simulink model "NeuralNetworkAdaptiveControl_Example"  (R2019a)
settings: Solver=VariableStepAuto  StartTime=0.0  StopTime=10.0  RelTol=1e-3
InitFcn:
  | ini_file
values from neighbouring files (symbols this model uses):
  gamma = 3    [ini_file_HW.m]
  wn = 3    [ini_file_HW.m]
  zeta = 1    [ini_file_HW.m]
undefined symbols (not defined in the file or in its folder): sigbuilder_block
settings Model: Creator=0629w  LastModifiedBy=0629w

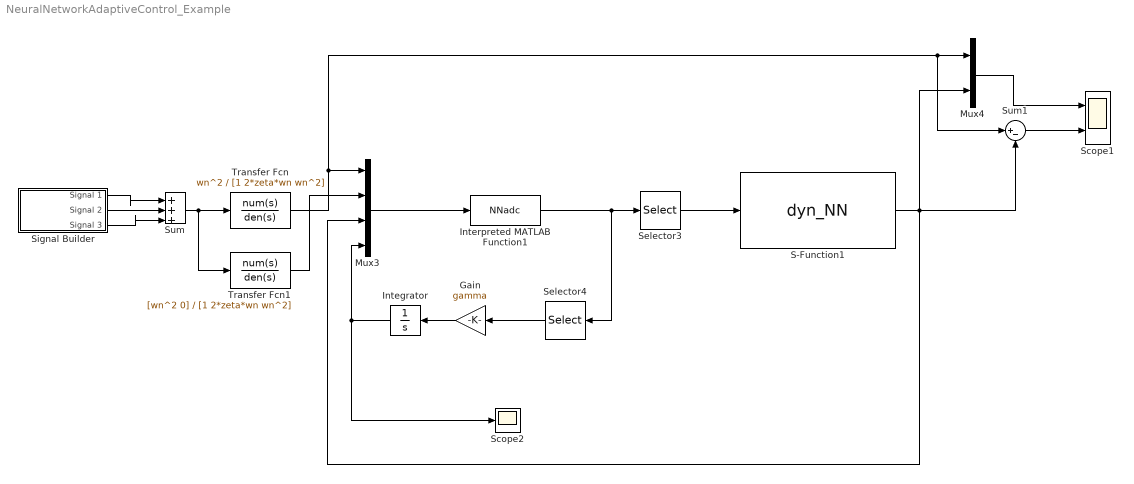
== system NeuralNetworkAdaptiveControl_Example ==
  Gain : Gain  Gain=gamma
  Integrator : Integrator
  Interpreted MATLAB Function1 : MATLABFcn  MATLABFcn=NNadc  OutputDimensions=3
  Mux3 : Mux
  Mux4 : Mux  Inputs=2
  S-Function1 : S-Function  FunctionName=dyn_NN  SFunctionDeploymentMode=off  EnableBusSupport=off
  Scope1 : Scope  NumInputPorts=2
  Scope2 : Scope
  Selector3 : Selector  InputPortWidth=3  IndexOptions=Index vector (dialog)  Indices=[1]  OutputSizes=1
  Selector4 : Selector  InputPortWidth=3  IndexOptions=Index vector (dialog)  Indices=[2 3]  OutputSizes=1
  Signal Builder : Subsystem  Tag=STV Subsys  LoadFcn=sigbuilder_block('load');  StartFcn=sigbuilder_block('start');  StopFcn=sigbuilder_block('stop');  ClipboardFcn=sigbuilder_block('clipboard');  mask(Sigbuilder block){tuvar=[0:10]}
      mask help: Simulink:masks:SigbuilderBlock_MD
      mask init:
      | if ~strcmp(get_param(bdroot(gcbh),'SimulationStatus'),'stopped') tuvar = sigbuilder_block('maskInit'); end
      settings: CopyFcn=sigbuilder_block('copy');  DeleteFcn=sigbuilder_block('delete');  ModelCloseFcn=sigbuilder_block('modelClose');  PreSaveFcn=sigbuilder_block('preSave');  PauseFcn=sigbuilder_block('pause');  ContinueFcn=sigbuilder_block('continue');  NameChangeFcn=sigbuilder_block('namechange');  OpenFcn=sigbuilder_block('open',[-192 38.25 1188 545.25 ]);  CloseFcn=sigbuilder_block('close');
      mask Display: plot(0, 0, 100, 100,[2, 2, 32, 32, 2], [68, 8, 8, 68, 68],[32, 2], [38, 38], [32, 19, 2],[53, 60, 44], [32, 17, 17, 2],[16, 16, 31, 31]);txt = getActiveGroup(gcbh);text(2, 100, txt,'verticalAlignment', 'top');
  Sum : Sum  Inputs=|+++
  Sum1 : Sum  Inputs=|+-
  Transfer Fcn : TransferFcn  Numerator=wn^2  Denominator=[1 2*zeta*wn wn^2]
  Transfer Fcn1 : TransferFcn  Numerator=[wn^2 0]  Denominator=[1 2*zeta*wn wn^2]
  wires:
  Mux4/1 -> Scope1/1
  Integrator/1 -> Scope2/1, Mux3/4
  Gain/1 -> Integrator/1
  Interpreted MATLAB Function1/1 -> Selector3/1, Selector4/1
  Selector3/1 -> S-Function1/1
  Selector4/1 -> Gain/1
  Mux3/1 -> Interpreted MATLAB Function1/1
  Signal Builder/1(Signal 1) -> Sum/1
  Signal Builder/2(Signal 2) -> Sum/2
  Signal Builder/3(Signal 3) -> Sum/3
  Sum/1 -> Transfer Fcn1/1, Transfer Fcn/1
  Transfer Fcn/1 -> Sum1/1, Mux4/1, Mux3/1
  Transfer Fcn1/1 -> Mux3/2
  S-Function1/1 -> Sum1/2, Mux3/3, Mux4/2
  Sum1/1 -> Scope1/2

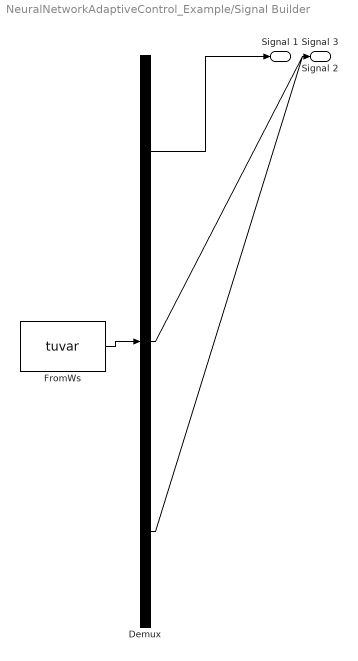
== system NeuralNetworkAdaptiveControl_Example/Signal Builder ==
  Demux : Demux  Tag=STV Demux  Outputs=3
  FromWs : FromWorkspace  Tag=STV FromWs  VariableName=tuvar  SampleTime=0
      SigBuilderData=|
      | common.afterFinalStr = 'Extrapolate'
      | common.sampleTime = 0
      | dataSet.timeRange = [0 10]
      | dataSet.name = 'Group 1'
      | sbobj.Groups.Name = 'Group 1'
      | sbobj.Groups.Signals(1).Name = 'Signal 1'
      | sbobj.Groups.Signals(1).XData = [0 4 4 6 6 10]
      | sbobj.Groups.Signals(1).YData = [-0.4 -0.4 0 0 0.6 0.6]
      | sbobj.Groups.Signals(2).Name = 'Signal 2'
      | sbobj.Groups.Signals(2).XData = [0 4 4 6 6 10]
      | sbobj.Groups.Signals(2).YData = [0 0.71 0.89 1 0.4 0]
      | sbobj.Groups.Signals(3).Name = 'Signal 3'
      | sbobj.Groups.Signals(3).XData = [0 10]
      | sbobj.Groups.Signals(3).YData = [0.98 0.98]
  Signal 1 : Outport  Tag=STV Outport
  Signal 2 : Outport  Tag=STV Outport  Port=2
  Signal 3 : Outport  Tag=STV Outport  Port=3
  wires:
  Demux/1 -> Signal 1/1
  FromWs/1 -> Demux/1
  Demux/2 -> Signal 2/1
  Demux/3 -> Signal 3/1
